simulink model "ReceiveAndSend_2018b"  (R2022a)
settings: Solver=VariableStepAuto  StartTime=0.0  StopTime=inf  RelTol=1e-3
libraries: instrumentseriallib x3
settings Model: Creator=NRPU  LastModifiedBy=NRPU
settings SolverCC: AlgebraicLoopSolver=TrustRegion
settings DebuggingCC: ArithmeticOperatorsInVariantConditions=warning
settings SFSimCC: CustomCodeUndefinedFunction=UseInterfaceOnly

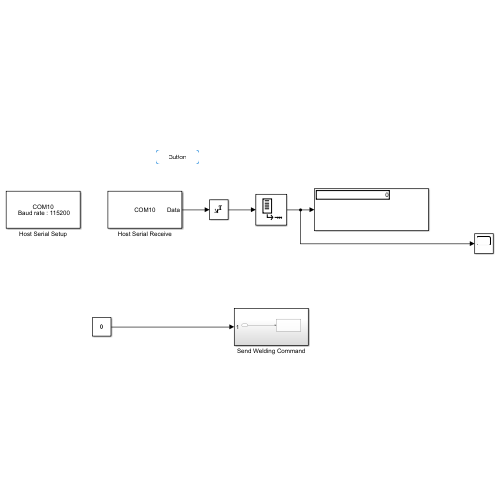
[thumbnail: Simulink's stored preview of the top-level diagram]
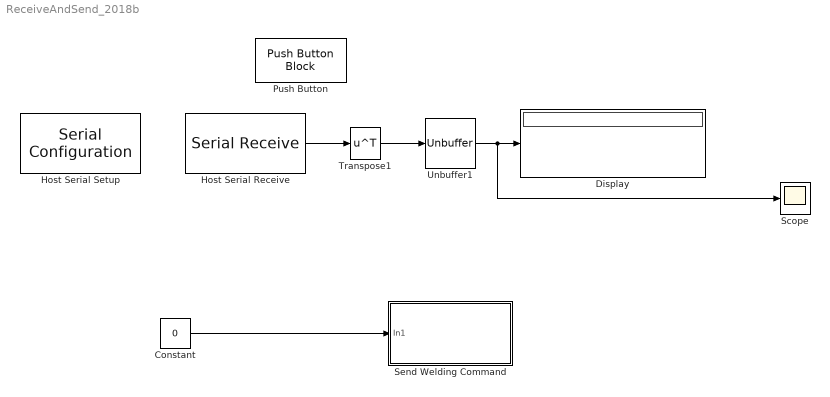
== system ReceiveAndSend_2018b ==
  Constant : Constant  Value=0  OutDataTypeStr=uint16
  Display : Display
  Host Serial Receive : instrumentseriallib/Serial Receive  PortSel=COM10  Port=COM10  ComPort=COM10  DataType=int32  SaveDataType=uint8  ToggleHeader=on  Header='SSSS'  ToggleTerminator=on  Terminator=Custom terminator  CustomTerminator='EEEE'  InputFormat=Row major  ToggleDataSize=on  DataSize=[1 1200]  EnableBlockingMode=on  ActionDataUnavailable=Output last received value  ActionWhenDataUnavailable=Output last received value  CustomValue=0  SampleTime=1  SimulateUsing=Interpreted execution  BlockInModel=on  aMode=5
      settings: SourceProductBaseCode=OT,IC,MT
  Host Serial Setup : instrumentseriallib/Serial Configuration  Priority=-99  PortSel=COM10  Port=COM10  ComPort=COM10  BaudRate=115200  DataBits=8  Parity=none  StopBits=1  ByteOrder=little-endian  FlowControl=none  Timeout=2  SimulateUsing=Interpreted execution  BlockInModel=on  aMode=5
      settings: SourceProductBaseCode=OT,IC,MT
  Push Button : PushButtonBlock  OffValue=0.000000
  Scope : Scope
  Send Welding Command : Subsystem
  Transpose1 : Math  Operator=transpose  SignedPower=on
  Unbuffer1 : Unbuffer
  wires:
  Transpose1/1 -> Unbuffer1/1
  Host Serial Receive/1 -> Transpose1/1
  Unbuffer1/1 -> Scope/1, Display/1
  Constant/1 -> Send Welding Command/1(In1)

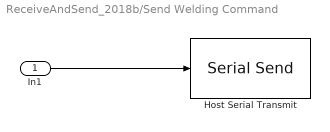
== system ReceiveAndSend_2018b/Send Welding Command ==
  In1 : Inport
  Host Serial Transmit : instrumentseriallib/Serial Send  PortSel=COM10  Port=COM10  ComPort=COM10  Header='S'  Terminator=Custom terminator  CustomTerminator='E'  EnableBlockingMode=on  SimulateUsing=Interpreted execution  BlockInModel=on  aMode=5
      settings: SourceProductBaseCode=OT,IC,MT
  wires:
  In1/1 -> Host Serial Transmit/1
